simulink model "Longitudinal_U"  (R2024b)
settings: Solver=VariableStepAuto  StartTime=0.0  StopTime=720  RelTol=1e-3
undefined symbols (not defined in the file): Kd_3, Ki_2, Ki_3, Ki_4, Ki_5, Kp_1, Kp_2, Kp_3, Kp_4, Kp_5
libraries: simulink x18, slpidlib x5
settings Model: Creator=GH-X-ST  LastModifiedBy=GH-X-ST

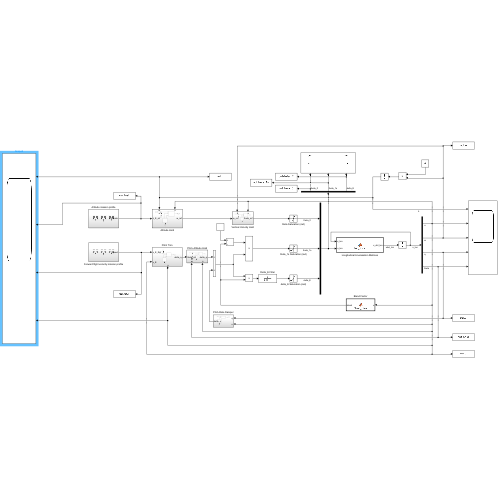
[thumbnail: Simulink's stored preview of the top-level diagram]
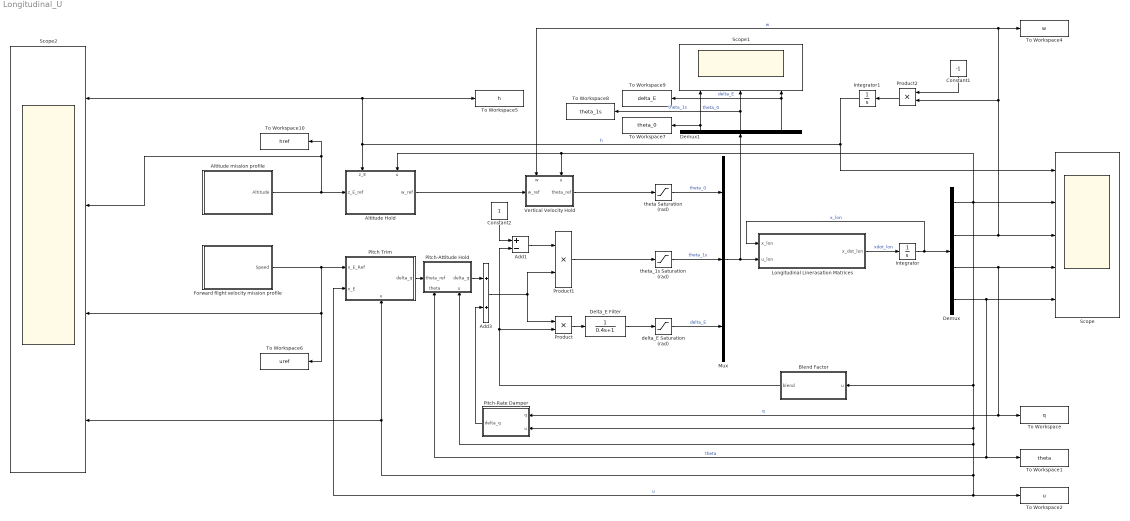
== system Longitudinal_U ==
  Add1 : Sum  Inputs=+-
  Add3 : Sum
  Altitude Hold : Subsystem
      settings: PortSchema="{\"entries\":[{\"content\":{\"sides\":[{\"content\":{\"connectorIds\":[\"In1\"]},\"type\":\"ConnectorPlacement.EquallySpacedRectSide\",\"uuid\":\"786fe27b-9d32-4a4b-ba58-745251b51298\"},{\"content\":{\"connectorIds\":[\"Out1\"],\"side\":\"RIGHT\"},\"type\":\"ConnectorPlacement.EquallySpacedRectSide\",\"uuid\":\"c3e63844-28f7-4108-b9b9-8f5ae49ef2b7\"},{\"content\":{\"connectorIds\":[\"In2\",\"In3\"],\"side\":\"TOP\"},\"type\":\"ConnectorPlacement.EquallySpacedRectSide\",\"uuid\":\"709e7f88-d3c1-4cf0-9a6f-fe71781ed8e6\"}]},\"type\":\"ConnectorPlacement.EquallySpacedConnector\",\"uuid\":\"916bac8a-d735-4a54-bfae-f4eae304bdce\"}],\"packageUris\":[\"http://schema.mathworks.com/mf0/Connector/R2020b\"],\"version\":\"1.0\"}"
  Altitude mission profile : Subsystem
  Blend Factor : MATLAB Function  TreatAsAtomicUnit=on
  Constant1 : Constant  Value=-1
  Constant2 : Constant
  Delta_E Filter : TransferFcn  Denominator=[0.4 1]
  Demux : Demux
  Demux1 : Demux  Outputs=3
  Forward flight velocity mission profile : Subsystem
  Integrator : Integrator  InitialCondition=[0.000000000001; 0; 0; 0]
  Integrator1 : Integrator  InitialCondition=135  ContinuousStateAttributes='h'
  Longitudinal Linerasation Matrices : MATLAB Function  TreatAsAtomicUnit=on
  Mux : Mux  Inputs=3
  Pitch Trim : Subsystem
      settings: PortSchema="{\"entries\":[{\"content\":{\"sides\":[{\"content\":{\"connectorIds\":[\"In1\",\"In2\"]},\"type\":\"ConnectorPlacement.EquallySpacedRectSide\",\"uuid\":\"87058170-54f3-49f3-bbe3-319f98d36a6e\"},{\"content\":{\"connectorIds\":[\"Out1\"],\"side\":\"RIGHT\"},\"type\":\"ConnectorPlacement.EquallySpacedRectSide\",\"uuid\":\"504f7628-6ca7-48d8-902d-2d0a87ee545b\"},{\"content\":{\"side\":\"TOP\"},\"type\":\"ConnectorPlacement.EquallySpacedRectSide\",\"uuid\":\"0adfc2aa-d413-4184-8660-649e124bfc66\"},{\"content\":{\"connectorIds\":[\"In3\"],\"side\":\"BOTTOM\"},\"type\":\"ConnectorPlacement.EquallySpacedRectSide\",\"uuid\":\"db6c614d-9f31-4390-b799-cc5d953a9def\"}]},\"type\":\"ConnectorPlacement.EquallySpacedConnector\",\"uuid\":\"6825786d-d4a2-4d28-866f-fdc5057e89d5\"}],\"packageUris\":[\"http://schema.mathworks.com/mf0/Connector/R2020b\"],\"version\":\"1.0\"}"
  Pitch-Attitude Hold : Subsystem
      settings: PortSchema="{\"entries\":[{\"content\":{\"sides\":[{\"content\":{\"connectorIds\":[\"In1\"]},\"type\":\"ConnectorPlacement.EquallySpacedRectSide\",\"uuid\":\"6ee333b9-9b69-42fd-975a-4580f9624540\"},{\"content\":{\"connectorIds\":[\"Out1\"],\"side\":\"RIGHT\"},\"type\":\"ConnectorPlacement.EquallySpacedRectSide\",\"uuid\":\"6a43d978-a0a5-4636-bfdb-b097e996a039\"},{\"content\":{\"side\":\"TOP\"},\"type\":\"ConnectorPlacement.EquallySpacedRectSide\",\"uuid\":\"00f937d1-ecc9-42d4-adf8-d8f1b79c75a6\"},{\"content\":{\"connectorIds\":[\"In2\",\"In3\"],\"side\":\"BOTTOM\"},\"type\":\"ConnectorPlacement.EquallySpacedRectSide\",\"uuid\":\"809403f9-594f-4491-8a7d-ee0f8643f57e\"}]},\"type\":\"ConnectorPlacement.EquallySpacedConnector\",\"uuid\":\"362aafbc-ebc0-4bb3-8c4e-be284a8bc83f\"}],\"packageUris\":[\"http://schema.mathworks.com/mf0/Connector/R2020b\"],\"version\":\"1.0\"}"
  Pitch-Rate Damper : Subsystem
  Product : Product
  Product1 : Product
  Product2 : Product
  Scope : Scope  NumInputPorts=5
  Scope1 : Scope  NumInputPorts=3
  Scope2 : Scope  NumInputPorts=4
  To Workspace : ToWorkspace  VariableName=q  SaveFormat=Timeseries  SampleTime=-1
  To Workspace1 : ToWorkspace  VariableName=theta  SaveFormat=Timeseries  SampleTime=-1
  To Workspace10 : ToWorkspace  VariableName=href  SaveFormat=Timeseries  SampleTime=-1
  To Workspace2 : ToWorkspace  VariableName=u  SaveFormat=Timeseries  SampleTime=-1
  To Workspace4 : ToWorkspace  VariableName=w  SaveFormat=Timeseries  SampleTime=-1
  To Workspace5 : ToWorkspace  VariableName=h  SaveFormat=Timeseries  SampleTime=-1
  To Workspace6 : ToWorkspace  VariableName=uref  SaveFormat=Timeseries  SampleTime=-1
  To Workspace7 : ToWorkspace  VariableName=theta_0  SaveFormat=Timeseries  SampleTime=-1
  To Workspace8 : ToWorkspace  VariableName=theta_1s  SaveFormat=Timeseries  SampleTime=-1
  To Workspace9 : ToWorkspace  VariableName=delta_E  SaveFormat=Timeseries  SampleTime=-1
  Vertical Velocity Hold : Subsystem
      settings: PortSchema="{\"entries\":[{\"content\":{\"sides\":[{\"content\":{\"connectorIds\":[\"In1\"]},\"type\":\"ConnectorPlacement.EquallySpacedRectSide\",\"uuid\":\"6ee333b9-9b69-42fd-975a-4580f9624540\"},{\"content\":{\"connectorIds\":[\"Out1\"],\"side\":\"RIGHT\"},\"type\":\"ConnectorPlacement.EquallySpacedRectSide\",\"uuid\":\"6a43d978-a0a5-4636-bfdb-b097e996a039\"},{\"content\":{\"connectorIds\":[\"In2\",\"In3\"],\"side\":\"TOP\"},\"type\":\"ConnectorPlacement.EquallySpacedRectSide\",\"uuid\":\"00f937d1-ecc9-42d4-adf8-d8f1b79c75a6\"},{\"content\":{\"side\":\"BOTTOM\"},\"type\":\"ConnectorPlacement.EquallySpacedRectSide\",\"uuid\":\"64d125d6-056c-4640-9df5-5340aaf5f7d1\"}]},\"type\":\"ConnectorPlacement.EquallySpacedConnector\",\"uuid\":\"362aafbc-ebc0-4bb3-8c4e-be284a8bc83f\"}],\"packageUris\":[\"http://schema.mathworks.com/mf0/Connector/R2020b\"],\"version\":\"1.0\"}"
  delta_E Saturation (rad) : Saturate  UpperLimit=deg2rad(11)  LowerLimit=deg2rad(-11)
  theta Saturation (rad) : Saturate  UpperLimit=deg2rad(+20)  LowerLimit=deg2rad(-6)
  theta_1s Saturation (rad) : Saturate  UpperLimit=deg2rad(6)  LowerLimit=deg2rad(-6)
  wires:
  Longitudinal Linerasation Matrices/1(x_dot_lon) -> Integrator/1  "xdot_lon"
  Integrator/1 -> Longitudinal Linerasation Matrices/1(x_lon), Demux/1  "x_lon"
  Demux/1 -> Altitude Hold/3(u), Vertical Velocity Hold/3(u), Scope/2, Blend Factor/1(u), Pitch-Attitude Hold/3(u), Pitch Trim/3(u), Scope2/4, To Workspace2/1, Pitch Trim/2(x_E), Pitch-Rate Damper/2(u)  "u"
  Demux/2 -> Vertical Velocity Hold/2(w), To Workspace4/1, Product2/2, Scope/3  "w"
  Demux/3 -> Scope/4, To Workspace/1, Pitch-Rate Damper/1(q)  "q"
  Demux/4 -> Scope/5, To Workspace1/1, Pitch-Attitude Hold/2(theta)  "theta"
  Blend Factor/1(blend) -> Add1/2, Product/2
  Pitch-Attitude Hold/1(delta_q) -> Add3/1
  Constant2/1 -> Add1/1
  Add1/1 -> Product1/1
  Mux/1 -> Demux1/1, Longitudinal Linerasation Matrices/2(u_lon)
  Demux1/3 -> To Workspace9/1, Scope1/3  "delta_E"
  Demux1/2 -> Scope1/2, To Workspace8/1  "theta_1s"
  Demux1/1 -> Scope1/1, To Workspace7/1  "theta_0"
  Product/1 -> Delta_E Filter/1
  Pitch-Rate Damper/1(delta_q) -> Add3/2
  Constant1/1 -> Product2/1
  Product2/1 -> Integrator1/1
  Integrator1/1 -> Scope/1, Altitude Hold/2(z_E), Scope2/1, To Workspace5/1  "h"
  Altitude Hold/1(w_ref) -> Vertical Velocity Hold/1(w_ref)
  Add3/1 -> Product1/2, Product/1
  Pitch Trim/1(delta_q) -> Pitch-Attitude Hold/1(theta_ref)
  Delta_E Filter/1 -> delta_E Saturation (rad)/1
  delta_E Saturation (rad)/1 -> Mux/3  "delta_E"
  theta_1s Saturation (rad)/1 -> Mux/2  "theta_1s"
  Product1/1 -> theta_1s Saturation (rad)/1
  Vertical Velocity Hold/1(theta_ref) -> theta Saturation (rad)/1
  theta Saturation (rad)/1 -> Mux/1  "theta_0"
  Altitude mission profile/1(Altitude) -> To Workspace10/1, Scope2/2, Altitude Hold/1(z_E_ref)
  Forward flight velocity mission profile/1(Speed) -> To Workspace6/1, Scope2/3, Pitch Trim/1(x_E_Ref)

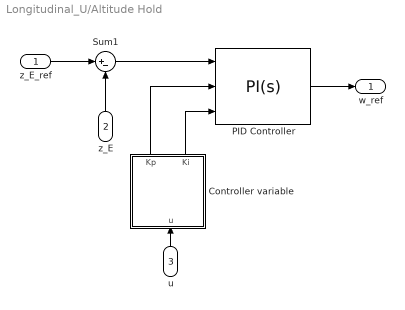
== system Longitudinal_U/Altitude Hold ==
  z_E_ref : Inport
  z_E : Inport  Port=2
  u : Inport  Port=3
  Controller variable : MATLAB Function  TreatAsAtomicUnit=on
  PID Controller : slpidlib/PID Controller  Controller=PI  Form=Parallel  TimeDomain=Continuous-time  UseExternalTs=off  SampleTime=-1  IntegratorMethod=Forward Euler  FilterMethod=Forward Euler  ControllerParametersSource=external  P=Kp_5  I=Ki_5  UseKiTs=off  D=0.005  UseExternalDerivativeSource=off  N=100  UseFilter=on  TunerSelectOption=Transfer Function Based (PID Tuner App)  InitialConditionSource=internal  InitialConditionForIntegrator=0  InitialConditionForFilter=0  DifferentiatorICPrevScaledInput=0  ExternalReset=none  TrackingMode=off  Kt=1  LimitOutput=on  SatLimitsSource=internal  UpperSaturationLimit=1  LowerSaturationLimit=-1  LinearizeAsGain=on  AntiWindupMode=none  Kb=1  LimitIntegrator=off  UpperIntegratorSaturationLimit=inf  LowerIntegratorSaturationLimit=-inf  POutMin=[]  POutMax=[]  IOutMin=[]  IOutMax=[]  DOutMin=[]  DOutMax=[]  NOutMin=[]  NOutMax=[]  SumOutMin=[]  SumOutMax=[]  SaturationOutMin=[]  SaturationOutMax=[]  PParamMin=[]  PParamMax=[]  IParamMin=[]  IParamMax=[]  DParamMin=[]  DParamMax=[]  NParamMin=[]  NParamMax=[]  KbParamMin=[]  KbParamMax=[]  KtParamMin=[]  KtParamMax=[]  KbOutMin=[]  KbOutMax=[]  KtOutMin=[]  KtOutMax=[]  IntegratorOutMin=[]  IntegratorOutMax=[]  FilterOutMin=[]  FilterOutMax=[]  SumI1OutMin=[]  SumI1OutMax=[]  SumI2OutMin=[]  SumI2OutMax=[]  SumI3OutMin=[]  SumI3OutMax=[]  SumI4OutMin=[]  SumI4OutMax=[]  SumDOutMin=[]  SumDOutMax=[]  DifferentiatorOutMin=[]  DifferentiatorOutMax=[]  FilterDiffOutCoefMin=[]  FilterDiffOutCoefMax=[]  ReciprocalOutMin=[]  ReciprocalOutMax=[]  SumDenOutMin=[]  SumDenOutMax=[]  SumNumOutMin=[]  SumNumOutMax=[]  DivideOutMin=[]  DivideOutMax=[]  UdiffTsProdOutMin=[]  UdiffTsProdOutMax=[]  NTsProdOutMin=[]  NTsProdOutMax=[]  UintegralTsProdOutMin=[]  UintegralTsProdOutMax=[]  UngainTsProdOutMin=[]  UngainTsProdOutMax=[]  ClampingZeroOutDataTypeStr=Inherit: Inherit via back propagation  ClampingZeroOutMin=[]  ClampingZeroOutMax=[]  FilterDenConstantOutDataTypeStr=Inherit: Inherit via back propagation  FilterDenConstantOutMin=[]  FilterDenConstantOutMax=[]  PCopyOutDataTypeStr=Inherit: Inherit via back propagation  PCopyOutMin=[]  PCopyOutMax=[]  NCopyOutDataTypeStr=Inherit: Inherit via back propagation  NCopyOutMin=[]  NCopyOutMax=[]  IntegratorContinuousStateAttributes=''  IntegratorStateMustResolveToSignalObject=off  IntegratorRTWStateStorageClass=Auto  FilterContinuousStateAttributes=''  FilterStateMustResolveToSignalObject=off  FilterRTWStateStorageClass=Auto  ParallelPVariant=ExternalParameters  IdealPVariant=Disabled  IVariant=ExternalParameters  DVariant=Disabled  IntegratorVariant=Continuous  SatVariant=Enabled  AWVariant=Passthrough  PCopyVariant=Disabled  TRVariant=Disabled  FdbkBlocksVariant=Forward  IdealPFdbkVariant=Disabled  SatFdbkVariant=Disabled  DerivativeFilterVariant=Disabled  NVariant=Disabled  NCopyVariant=Disabled_SignalSpec  FilterICVariant=Disabled  IntegratorICVariant=InternalICs  ExternalResetVariant=Disabled  TRSumVariant=Passthrough  SumFdbkVariant=Disabled  SumVariant=Sum_PI  TsampFilterVariant=InternalTs  TsampNgainVariant=Passthrough  TsampIntegralVariant=Disabled_SignalSpec  ExternalSaturationOutDataTypeStr=Inherit: Same as second input  DerivativeSourceVariant=Disabled  PreIntVariant=InternalPreInt
  Sum1 : Sum  Inputs=|+-
  w_ref : Outport
  wires:
  PID Controller/1 -> w_ref/1
  Sum1/1 -> PID Controller/1
  z_E_ref/1 -> Sum1/1
  z_E/1 -> Sum1/2
  u/1 -> Controller variable/1(u)
  Controller variable/1(Kp) -> PID Controller/2
  Controller variable/2(Ki) -> PID Controller/3

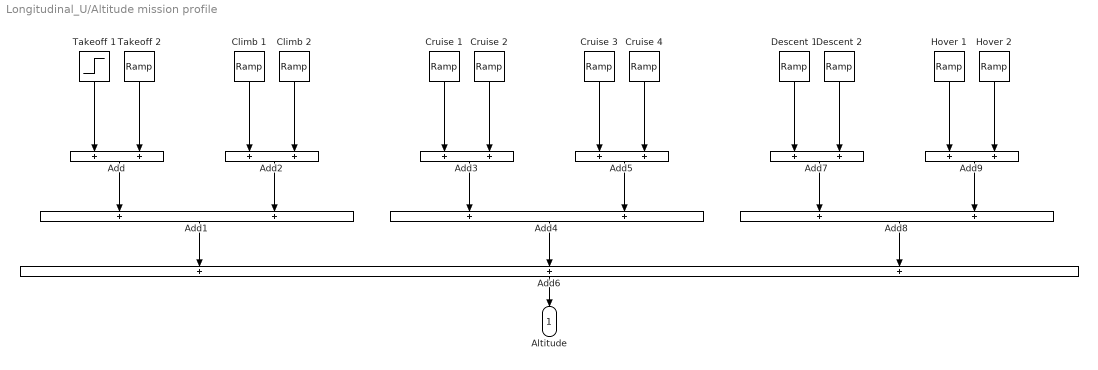
== system Longitudinal_U/Altitude mission profile ==
  Add{,1..5,7..9} (9 alike) : Sum
  Add6 : Sum  Inputs=+++
  Climb 1 : simulink/Sources/Ramp  slope=0.4  start=50  InitialOutput=0
  Climb 2 : simulink/Sources/Ramp  slope=-0.4  start=100  InitialOutput=0
  Cruise 1 : simulink/Sources/Ramp  slope=0.1  start=100  InitialOutput=0
  Cruise 2 : simulink/Sources/Ramp  slope=-0.1  start=200  InitialOutput=0
  Cruise 3 : simulink/Sources/Ramp  slope=0  start=200  InitialOutput=0
  Cruise 4 : simulink/Sources/Ramp  slope=0  start=350  InitialOutput=0
  Descent 1 : simulink/Sources/Ramp  slope=-12/70  start=350  InitialOutput=0
  Descent 2 : simulink/Sources/Ramp  slope=12/70  start=475  InitialOutput=0
  Hover 1 : simulink/Sources/Ramp  slope=0  start=475  InitialOutput=0
  Hover 2 : simulink/Sources/Ramp  slope=0  start=600  InitialOutput=0
  Takeoff 1 : Step  Time=0  Before=135  After=150  SampleTime=0
  Takeoff 2 : simulink/Sources/Ramp  slope=0  start=50  InitialOutput=0
  Altitude : Outport
  wires:
  Add1/1 -> Add6/1
  Climb 2/1 -> Add2/2
  Add4/1 -> Add6/2
  Climb 1/1 -> Add2/1
  Hover 1/1 -> Add9/1
  Add7/1 -> Add8/1
  Descent 1/1 -> Add7/1
  Add9/1 -> Add8/2
  Hover 2/1 -> Add9/2
  Add8/1 -> Add6/3
  Add2/1 -> Add1/2
  Add3/1 -> Add4/1
  Add5/1 -> Add4/2
  Cruise 2/1 -> Add3/2
  Cruise 4/1 -> Add5/2
  Cruise 1/1 -> Add3/1
  Cruise 3/1 -> Add5/1
  Descent 2/1 -> Add7/2
  Takeoff 2/1 -> Add/2
  Takeoff 1/1 -> Add/1
  Add/1 -> Add1/1
  Add6/1 -> Altitude/1

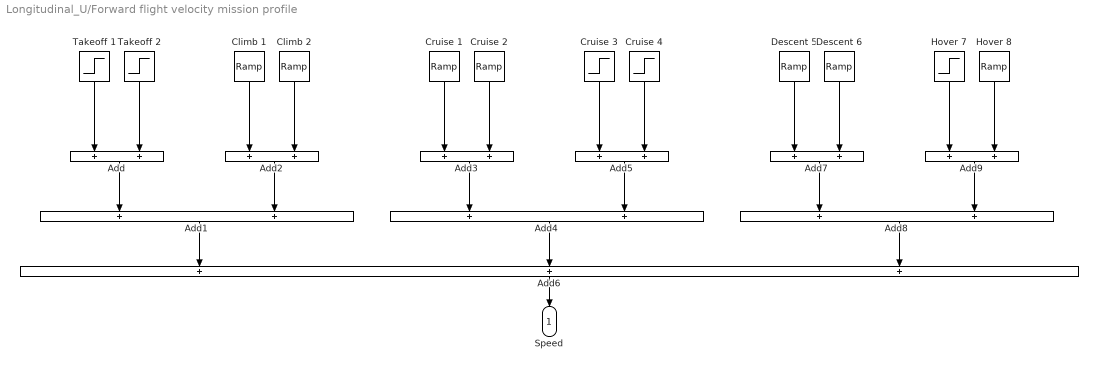
== system Longitudinal_U/Forward flight velocity mission profile ==
  Add{,1..5,7..9} (9 alike) : Sum
  Add6 : Sum  Inputs=+++
  Climb 1 : simulink/Sources/Ramp  slope=0.4  start=50  InitialOutput=0
  Climb 2 : simulink/Sources/Ramp  slope=-0.4  start=100  InitialOutput=0
  Cruise 1 : simulink/Sources/Ramp  slope=0  start=100  InitialOutput=0
  Cruise 2 : simulink/Sources/Ramp  slope=0  start=200  InitialOutput=0
  Cruise 3 : Step  Time=200  After=22  SampleTime=0
  Cruise 4 : Step  Time=350  After=-37  SampleTime=0
  Descent 5 : simulink/Sources/Ramp  slope=0  start=350  InitialOutput=0
  Descent 6 : simulink/Sources/Ramp  slope=0  start=475  InitialOutput=0
  Hover 7 : Step  Time=475  After=-35  SampleTime=0
  Hover 8 : simulink/Sources/Ramp  slope=0  start=600  InitialOutput=0
  Takeoff 1 : Step  Time=0  After=0  SampleTime=0
  Takeoff 2 : Step  Time=50  After=30  SampleTime=0
  Speed : Outport
  wires:
  Add6/1 -> Speed/1
  Add1/1 -> Add6/1
  Climb 2/1 -> Add2/2
  Add4/1 -> Add6/2
  Climb 1/1 -> Add2/1
  Add7/1 -> Add8/1
  Descent 5/1 -> Add7/1
  Add9/1 -> Add8/2
  Descent 6/1 -> Add7/2
  Hover 8/1 -> Add9/2
  Add8/1 -> Add6/3
  Add2/1 -> Add1/2
  Add3/1 -> Add4/1
  Add5/1 -> Add4/2
  Cruise 1/1 -> Add3/1
  Cruise 4/1 -> Add5/2
  Add/1 -> Add1/1
  Hover 7/1 -> Add9/1
  Takeoff 1/1 -> Add/1
  Takeoff 2/1 -> Add/2
  Cruise 3/1 -> Add5/1
  Cruise 2/1 -> Add3/2

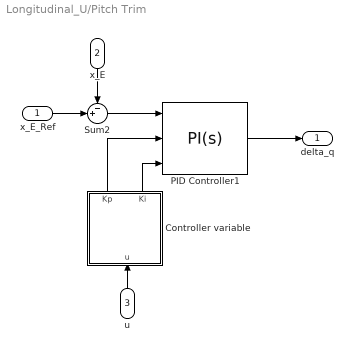
== system Longitudinal_U/Pitch Trim ==
  x_E_Ref : Inport
  x_E : Inport  Port=2
  u : Inport  Port=3
  Controller variable : MATLAB Function  TreatAsAtomicUnit=on
  PID Controller1 : slpidlib/PID Controller  Controller=PI  Form=Parallel  TimeDomain=Continuous-time  UseExternalTs=off  SampleTime=-1  IntegratorMethod=Forward Euler  FilterMethod=Forward Euler  ControllerParametersSource=external  P=Kp_3  I=Ki_3  UseKiTs=off  D=Kd_3  UseExternalDerivativeSource=off  N=100  UseFilter=on  TunerSelectOption=Transfer Function Based (PID Tuner App)  InitialConditionSource=internal  InitialConditionForIntegrator=0  InitialConditionForFilter=0  DifferentiatorICPrevScaledInput=0  ExternalReset=none  TrackingMode=off  Kt=1  LimitOutput=on  SatLimitsSource=internal  UpperSaturationLimit=1  LowerSaturationLimit=-1  LinearizeAsGain=on  AntiWindupMode=none  Kb=1  LimitIntegrator=off  UpperIntegratorSaturationLimit=inf  LowerIntegratorSaturationLimit=-inf  POutMin=[]  POutMax=[]  IOutMin=[]  IOutMax=[]  DOutMin=[]  DOutMax=[]  NOutMin=[]  NOutMax=[]  SumOutMin=[]  SumOutMax=[]  SaturationOutMin=[]  SaturationOutMax=[]  PParamMin=[]  PParamMax=[]  IParamMin=[]  IParamMax=[]  DParamMin=[]  DParamMax=[]  NParamMin=[]  NParamMax=[]  KbParamMin=[]  KbParamMax=[]  KtParamMin=[]  KtParamMax=[]  KbOutMin=[]  KbOutMax=[]  KtOutMin=[]  KtOutMax=[]  IntegratorOutMin=[]  IntegratorOutMax=[]  FilterOutMin=[]  FilterOutMax=[]  SumI1OutMin=[]  SumI1OutMax=[]  SumI2OutMin=[]  SumI2OutMax=[]  SumI3OutMin=[]  SumI3OutMax=[]  SumI4OutMin=[]  SumI4OutMax=[]  SumDOutMin=[]  SumDOutMax=[]  DifferentiatorOutMin=[]  DifferentiatorOutMax=[]  FilterDiffOutCoefMin=[]  FilterDiffOutCoefMax=[]  ReciprocalOutMin=[]  ReciprocalOutMax=[]  SumDenOutMin=[]  SumDenOutMax=[]  SumNumOutMin=[]  SumNumOutMax=[]  DivideOutMin=[]  DivideOutMax=[]  UdiffTsProdOutMin=[]  UdiffTsProdOutMax=[]  NTsProdOutMin=[]  NTsProdOutMax=[]  UintegralTsProdOutMin=[]  UintegralTsProdOutMax=[]  UngainTsProdOutMin=[]  UngainTsProdOutMax=[]  ClampingZeroOutDataTypeStr=Inherit: Inherit via back propagation  ClampingZeroOutMin=[]  ClampingZeroOutMax=[]  FilterDenConstantOutDataTypeStr=Inherit: Inherit via back propagation  FilterDenConstantOutMin=[]  FilterDenConstantOutMax=[]  PCopyOutDataTypeStr=Inherit: Inherit via back propagation  PCopyOutMin=[]  PCopyOutMax=[]  NCopyOutDataTypeStr=Inherit: Inherit via back propagation  NCopyOutMin=[]  NCopyOutMax=[]  IntegratorContinuousStateAttributes=''  IntegratorStateMustResolveToSignalObject=off  IntegratorRTWStateStorageClass=Auto  FilterContinuousStateAttributes=''  FilterStateMustResolveToSignalObject=off  FilterRTWStateStorageClass=Auto  ParallelPVariant=ExternalParameters  IdealPVariant=Disabled  IVariant=ExternalParameters  DVariant=Disabled  IntegratorVariant=Continuous  SatVariant=Enabled  AWVariant=Passthrough  PCopyVariant=Disabled  TRVariant=Disabled  FdbkBlocksVariant=Forward  IdealPFdbkVariant=Disabled  SatFdbkVariant=Disabled  DerivativeFilterVariant=Disabled  NVariant=Disabled  NCopyVariant=Disabled_SignalSpec  FilterICVariant=Disabled  IntegratorICVariant=InternalICs  ExternalResetVariant=Disabled  TRSumVariant=Passthrough  SumFdbkVariant=Disabled  SumVariant=Sum_PI  TsampFilterVariant=InternalTs  TsampNgainVariant=Passthrough  TsampIntegralVariant=Disabled_SignalSpec  ExternalSaturationOutDataTypeStr=Inherit: Same as second input  DerivativeSourceVariant=Disabled  PreIntVariant=InternalPreInt
  Sum2 : Sum  Inputs=-+|
  delta_q : Outport
  wires:
  x_E/1 -> Sum2/1
  x_E_Ref/1 -> Sum2/2
  PID Controller1/1 -> delta_q/1
  Sum2/1 -> PID Controller1/1
  u/1 -> Controller variable/1(u)
  Controller variable/1(Kp) -> PID Controller1/2
  Controller variable/2(Ki) -> PID Controller1/3

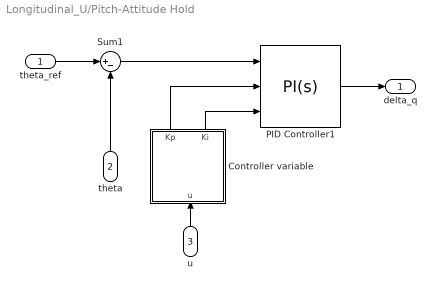
== system Longitudinal_U/Pitch-Attitude Hold ==
  theta_ref : Inport
  theta : Inport  Port=2
  u : Inport  Port=3
  Controller variable : MATLAB Function  TreatAsAtomicUnit=on
  PID Controller1 : slpidlib/PID Controller  Controller=PI  Form=Parallel  TimeDomain=Continuous-time  UseExternalTs=off  SampleTime=-1  IntegratorMethod=Forward Euler  FilterMethod=Forward Euler  ControllerParametersSource=external  P=Kp_2  I=Ki_2  UseKiTs=off  D=0.005  UseExternalDerivativeSource=on  N=100  UseFilter=on  TunerSelectOption=Transfer Function Based (PID Tuner App)  InitialConditionSource=internal  InitialConditionForIntegrator=0  InitialConditionForFilter=0  DifferentiatorICPrevScaledInput=0  ExternalReset=none  TrackingMode=off  Kt=1  LimitOutput=on  SatLimitsSource=internal  UpperSaturationLimit=1  LowerSaturationLimit=-1  LinearizeAsGain=on  AntiWindupMode=none  Kb=1  LimitIntegrator=off  UpperIntegratorSaturationLimit=inf  LowerIntegratorSaturationLimit=-inf  POutMin=[]  POutMax=[]  IOutMin=[]  IOutMax=[]  DOutMin=[]  DOutMax=[]  NOutMin=[]  NOutMax=[]  SumOutMin=[]  SumOutMax=[]  SaturationOutMin=[]  SaturationOutMax=[]  PParamMin=[]  PParamMax=[]  IParamMin=[]  IParamMax=[]  DParamMin=[]  DParamMax=[]  NParamMin=[]  NParamMax=[]  KbParamMin=[]  KbParamMax=[]  KtParamMin=[]  KtParamMax=[]  KbOutMin=[]  KbOutMax=[]  KtOutMin=[]  KtOutMax=[]  IntegratorOutMin=[]  IntegratorOutMax=[]  FilterOutMin=[]  FilterOutMax=[]  SumI1OutMin=[]  SumI1OutMax=[]  SumI2OutMin=[]  SumI2OutMax=[]  SumI3OutMin=[]  SumI3OutMax=[]  SumI4OutMin=[]  SumI4OutMax=[]  SumDOutMin=[]  SumDOutMax=[]  DifferentiatorOutMin=[]  DifferentiatorOutMax=[]  FilterDiffOutCoefMin=[]  FilterDiffOutCoefMax=[]  ReciprocalOutMin=[]  ReciprocalOutMax=[]  SumDenOutMin=[]  SumDenOutMax=[]  SumNumOutMin=[]  SumNumOutMax=[]  DivideOutMin=[]  DivideOutMax=[]  UdiffTsProdOutMin=[]  UdiffTsProdOutMax=[]  NTsProdOutMin=[]  NTsProdOutMax=[]  UintegralTsProdOutMin=[]  UintegralTsProdOutMax=[]  UngainTsProdOutMin=[]  UngainTsProdOutMax=[]  ClampingZeroOutDataTypeStr=Inherit: Inherit via back propagation  ClampingZeroOutMin=[]  ClampingZeroOutMax=[]  FilterDenConstantOutDataTypeStr=Inherit: Inherit via back propagation  FilterDenConstantOutMin=[]  FilterDenConstantOutMax=[]  PCopyOutDataTypeStr=Inherit: Inherit via back propagation  PCopyOutMin=[]  PCopyOutMax=[]  NCopyOutDataTypeStr=Inherit: Inherit via back propagation  NCopyOutMin=[]  NCopyOutMax=[]  IntegratorContinuousStateAttributes=''  IntegratorStateMustResolveToSignalObject=off  IntegratorRTWStateStorageClass=Auto  FilterContinuousStateAttributes=''  FilterStateMustResolveToSignalObject=off  FilterRTWStateStorageClass=Auto  ParallelPVariant=ExternalParameters  IdealPVariant=Disabled  IVariant=ExternalParameters  DVariant=Disabled  IntegratorVariant=Continuous  SatVariant=Enabled  AWVariant=Passthrough  PCopyVariant=Disabled  TRVariant=Disabled  FdbkBlocksVariant=Forward  IdealPFdbkVariant=Disabled  SatFdbkVariant=Disabled  DerivativeFilterVariant=Disabled  NVariant=Passthrough  NCopyVariant=Disabled_SignalSpec  FilterICVariant=Disabled  IntegratorICVariant=InternalICs  ExternalResetVariant=Disabled  TRSumVariant=Passthrough  SumFdbkVariant=Disabled  SumVariant=Sum_PI  TsampFilterVariant=InternalTs  TsampNgainVariant=Passthrough  TsampIntegralVariant=Disabled_SignalSpec  ExternalSaturationOutDataTypeStr=Inherit: Same as second input  DerivativeSourceVariant=Disabled  PreIntVariant=InternalPreInt
  Sum1 : Sum  Inputs=|+-
  delta_q : Outport
  wires:
  PID Controller1/1 -> delta_q/1
  theta_ref/1 -> Sum1/1
  theta/1 -> Sum1/2
  Sum1/1 -> PID Controller1/1
  Controller variable/1(Kp) -> PID Controller1/2
  Controller variable/2(Ki) -> PID Controller1/3
  u/1 -> Controller variable/1(u)

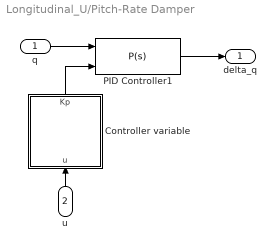
== system Longitudinal_U/Pitch-Rate Damper ==
  q : Inport
  u : Inport  Port=2
  Controller variable : MATLAB Function  TreatAsAtomicUnit=on
  PID Controller1 : slpidlib/PID Controller  Controller=P  Form=Parallel  TimeDomain=Continuous-time  UseExternalTs=off  SampleTime=-1  IntegratorMethod=Forward Euler  FilterMethod=Forward Euler  ControllerParametersSource=external  P=Kp_1  I=0.005  UseKiTs=off  D=0.005  UseExternalDerivativeSource=on  N=100  UseFilter=on  TunerSelectOption=Transfer Function Based (PID Tuner App)  InitialConditionSource=internal  InitialConditionForIntegrator=0  InitialConditionForFilter=0  DifferentiatorICPrevScaledInput=0  ExternalReset=none  TrackingMode=off  Kt=1  LimitOutput=on  SatLimitsSource=internal  UpperSaturationLimit=1  LowerSaturationLimit=-1  LinearizeAsGain=on  AntiWindupMode=none  Kb=1  LimitIntegrator=off  UpperIntegratorSaturationLimit=inf  LowerIntegratorSaturationLimit=-inf  POutMin=[]  POutMax=[]  IOutMin=[]  IOutMax=[]  DOutMin=[]  DOutMax=[]  NOutMin=[]  NOutMax=[]  SumOutMin=[]  SumOutMax=[]  SaturationOutMin=[]  SaturationOutMax=[]  PParamMin=[]  PParamMax=[]  IParamMin=[]  IParamMax=[]  DParamMin=[]  DParamMax=[]  NParamMin=[]  NParamMax=[]  KbParamMin=[]  KbParamMax=[]  KtParamMin=[]  KtParamMax=[]  KbOutMin=[]  KbOutMax=[]  KtOutMin=[]  KtOutMax=[]  IntegratorOutMin=[]  IntegratorOutMax=[]  FilterOutMin=[]  FilterOutMax=[]  SumI1OutMin=[]  SumI1OutMax=[]  SumI2OutMin=[]  SumI2OutMax=[]  SumI3OutMin=[]  SumI3OutMax=[]  SumI4OutMin=[]  SumI4OutMax=[]  SumDOutMin=[]  SumDOutMax=[]  DifferentiatorOutMin=[]  DifferentiatorOutMax=[]  FilterDiffOutCoefMin=[]  FilterDiffOutCoefMax=[]  ReciprocalOutMin=[]  ReciprocalOutMax=[]  SumDenOutMin=[]  SumDenOutMax=[]  SumNumOutMin=[]  SumNumOutMax=[]  DivideOutMin=[]  DivideOutMax=[]  UdiffTsProdOutMin=[]  UdiffTsProdOutMax=[]  NTsProdOutMin=[]  NTsProdOutMax=[]  UintegralTsProdOutMin=[]  UintegralTsProdOutMax=[]  UngainTsProdOutMin=[]  UngainTsProdOutMax=[]  ClampingZeroOutDataTypeStr=Inherit: Inherit via back propagation  ClampingZeroOutMin=[]  ClampingZeroOutMax=[]  FilterDenConstantOutDataTypeStr=Inherit: Inherit via back propagation  FilterDenConstantOutMin=[]  FilterDenConstantOutMax=[]  PCopyOutDataTypeStr=Inherit: Inherit via back propagation  PCopyOutMin=[]  PCopyOutMax=[]  NCopyOutDataTypeStr=Inherit: Inherit via back propagation  NCopyOutMin=[]  NCopyOutMax=[]  IntegratorContinuousStateAttributes=''  IntegratorStateMustResolveToSignalObject=off  IntegratorRTWStateStorageClass=Auto  FilterContinuousStateAttributes=''  FilterStateMustResolveToSignalObject=off  FilterRTWStateStorageClass=Auto  ParallelPVariant=ExternalParameters  IdealPVariant=Disabled  IVariant=Disabled  DVariant=Disabled  IntegratorVariant=Disabled  SatVariant=Enabled  AWVariant=Disabled  PCopyVariant=Disabled  TRVariant=Disabled  FdbkBlocksVariant=Forward  IdealPFdbkVariant=Disabled  SatFdbkVariant=Disabled  DerivativeFilterVariant=Disabled  NVariant=Passthrough  NCopyVariant=Disabled_SignalSpec  FilterICVariant=Disabled  IntegratorICVariant=Disabled  ExternalResetVariant=Disabled  TRSumVariant=Passthrough  SumFdbkVariant=Disabled  SumVariant=Passthrough_P  TsampFilterVariant=InternalTs  TsampNgainVariant=Passthrough  TsampIntegralVariant=Disabled_SignalSpec  ExternalSaturationOutDataTypeStr=Inherit: Same as second input  DerivativeSourceVariant=Disabled  PreIntVariant=InternalPreInt
  delta_q : Outport
  wires:
  PID Controller1/1 -> delta_q/1
  q/1 -> PID Controller1/1
  Controller variable/1(Kp) -> PID Controller1/2
  u/1 -> Controller variable/1(u)

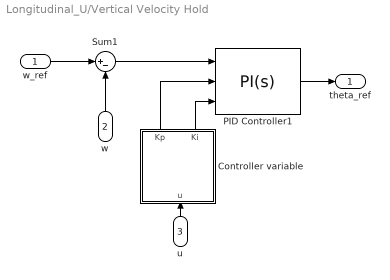
== system Longitudinal_U/Vertical Velocity Hold ==
  w_ref : Inport
  w : Inport  Port=2
  u : Inport  Port=3
  Controller variable : MATLAB Function  TreatAsAtomicUnit=on
  PID Controller1 : slpidlib/PID Controller  Controller=PI  Form=Parallel  TimeDomain=Continuous-time  UseExternalTs=off  SampleTime=-1  IntegratorMethod=Forward Euler  FilterMethod=Forward Euler  ControllerParametersSource=external  P=Kp_4  I=Ki_4  UseKiTs=off  D=0.005  UseExternalDerivativeSource=on  N=100  UseFilter=on  TunerSelectOption=Transfer Function Based (PID Tuner App)  InitialConditionSource=internal  InitialConditionForIntegrator=0  InitialConditionForFilter=0  DifferentiatorICPrevScaledInput=0  ExternalReset=none  TrackingMode=off  Kt=1  LimitOutput=on  SatLimitsSource=internal  UpperSaturationLimit=1  LowerSaturationLimit=-1  LinearizeAsGain=on  AntiWindupMode=none  Kb=1  LimitIntegrator=off  UpperIntegratorSaturationLimit=inf  LowerIntegratorSaturationLimit=-inf  POutMin=[]  POutMax=[]  IOutMin=[]  IOutMax=[]  DOutMin=[]  DOutMax=[]  NOutMin=[]  NOutMax=[]  SumOutMin=[]  SumOutMax=[]  SaturationOutMin=[]  SaturationOutMax=[]  PParamMin=[]  PParamMax=[]  IParamMin=[]  IParamMax=[]  DParamMin=[]  DParamMax=[]  NParamMin=[]  NParamMax=[]  KbParamMin=[]  KbParamMax=[]  KtParamMin=[]  KtParamMax=[]  KbOutMin=[]  KbOutMax=[]  KtOutMin=[]  KtOutMax=[]  IntegratorOutMin=[]  IntegratorOutMax=[]  FilterOutMin=[]  FilterOutMax=[]  SumI1OutMin=[]  SumI1OutMax=[]  SumI2OutMin=[]  SumI2OutMax=[]  SumI3OutMin=[]  SumI3OutMax=[]  SumI4OutMin=[]  SumI4OutMax=[]  SumDOutMin=[]  SumDOutMax=[]  DifferentiatorOutMin=[]  DifferentiatorOutMax=[]  FilterDiffOutCoefMin=[]  FilterDiffOutCoefMax=[]  ReciprocalOutMin=[]  ReciprocalOutMax=[]  SumDenOutMin=[]  SumDenOutMax=[]  SumNumOutMin=[]  SumNumOutMax=[]  DivideOutMin=[]  DivideOutMax=[]  UdiffTsProdOutMin=[]  UdiffTsProdOutMax=[]  NTsProdOutMin=[]  NTsProdOutMax=[]  UintegralTsProdOutMin=[]  UintegralTsProdOutMax=[]  UngainTsProdOutMin=[]  UngainTsProdOutMax=[]  ClampingZeroOutDataTypeStr=Inherit: Inherit via back propagation  ClampingZeroOutMin=[]  ClampingZeroOutMax=[]  FilterDenConstantOutDataTypeStr=Inherit: Inherit via back propagation  FilterDenConstantOutMin=[]  FilterDenConstantOutMax=[]  PCopyOutDataTypeStr=Inherit: Inherit via back propagation  PCopyOutMin=[]  PCopyOutMax=[]  NCopyOutDataTypeStr=Inherit: Inherit via back propagation  NCopyOutMin=[]  NCopyOutMax=[]  IntegratorContinuousStateAttributes=''  IntegratorStateMustResolveToSignalObject=off  IntegratorRTWStateStorageClass=Auto  FilterContinuousStateAttributes=''  FilterStateMustResolveToSignalObject=off  FilterRTWStateStorageClass=Auto  ParallelPVariant=ExternalParameters  IdealPVariant=Disabled  IVariant=ExternalParameters  DVariant=Disabled  IntegratorVariant=Continuous  SatVariant=Enabled  AWVariant=Passthrough  PCopyVariant=Disabled  TRVariant=Disabled  FdbkBlocksVariant=Forward  IdealPFdbkVariant=Disabled  SatFdbkVariant=Disabled  DerivativeFilterVariant=Disabled  NVariant=Passthrough  NCopyVariant=Disabled_SignalSpec  FilterICVariant=Disabled  IntegratorICVariant=InternalICs  ExternalResetVariant=Disabled  TRSumVariant=Passthrough  SumFdbkVariant=Disabled  SumVariant=Sum_PI  TsampFilterVariant=InternalTs  TsampNgainVariant=Passthrough  TsampIntegralVariant=Disabled_SignalSpec  ExternalSaturationOutDataTypeStr=Inherit: Same as second input  DerivativeSourceVariant=Disabled  PreIntVariant=InternalPreInt
  Sum1 : Sum  Inputs=|+-
  theta_ref : Outport
  wires:
  PID Controller1/1 -> theta_ref/1
  Sum1/1 -> PID Controller1/1
  w_ref/1 -> Sum1/1
  w/1 -> Sum1/2
  u/1 -> Controller variable/1(u)
  Controller variable/1(Kp) -> PID Controller1/2
  Controller variable/2(Ki) -> PID Controller1/3

== matlab function Longitudinal_U/Pitch-Rate Damper/Controller variable ==
  data: Kp output; u input
function Kp = Find_K1(u)
% Author:
%   Hanchen Li (hl3422@ic.ac.uk)
%
% Inputs:
%   u         - Forward velocity (m/s)
%
% Outputs:
%  Kp

U = [10.01; 20; 40; 60; 72.0222222];

if abs(u) <= 40

    Kp = 25.3;

else

    u = abs(u);
    u = min(max(u, min(U)), max(U));
    
    Kp_s = [97.0 84.1 25.3 9.65 7.80];
    
    Kp =  interp1(U, Kp_s, u, 'pchip', 'extrap');
    
end

end

== matlab function Longitudinal_U/Longitudinal Linerasation Matrices ==
  data: x_lon input; u_lon input; x_dot_lon output
function x_dot_lon = Lon_linear(x_lon, u_lon)
% Author:
%   Hanchen Li (hl3422@ic.ac.uk)
%
% Inputs:
%   x_lon     - [u, w, q, theta]
%   u         - Forward velocity (m/s)
%   w         - Vertical velocity (m/s)
%   q         - Pitch rate (rad/s)
%   theta     - Euler pitch angle (rad)
%
%   u_lon     - [theta_0, theta_1s, delta_E]
%   theta_0   - Average rotor collective (rad)
%   theta_1s  - Longitudinal cyclic (rad)
%   delta_E   - Elevator deflection (rad)
%
% Outputs:
%   x_dot_lon - [u_dot, w_dot, q_dot, theta_dot]

%% 0 Extract Parameters
u     = x_lon(1);
% w     = x_lon(2);
% q     = x_lon(3);
% theta = x_lon(4);

% theta_0 = u_lon(1);
% theta_1s = u_lon(2);
% delta_E = u_lon(3);

%%  1 Initial parameters
U = [10.01; 20; 40; 60; 72.0222222];       % 5 break-points

A_lon_all = cat(3,...
[0.00797773730409901	0.0742775144324526	-1.21387619054530	-9.79666335749863;
-0.300981219236718	-1.37899711980971	10.9535968552343	-0.454094238238056;
0.0867879507802988	0.0518221856357636	-1.66200207187276	0;
0	0	0.999987703616044	0],...
[-0.0112549858980772	0.0371668055628924	-1.18927896465665	-9.80422222650819;
-0.133476123611587	-1.29584894245305	20.8981012783838	-0.0361550902372443;
0.0229512851532743	0.0212311520956117	-1.57834195971935	0;
0	0	0.999823172370649	0],...
[-0.00894644618554263	0.0320555490226915	-1.19654303458228	-9.78886874671681;
0.0177938328871363	-2.75625714952099	41.9669994347238	0.0565348232672847;
0.00544480361520019	0.0390031290231026	-1.68547625422026	0;
0	0	0.999701937133157	0],...
[-0.00115522776185373	0.0138477446845475	-1.25249222634898	-9.78189512322418;
0.129681745697496	-2.84658770249635	62.0992998719228	-0.370385725787514;
-6.84962619262734e-05	0.0554454638454316	-1.71412794300992	0;
0	0	0.999829013944947	0],...
[0.00198907487199834	0.00124807180451603	-1.31545814391634	-9.77936080280246;
0.208959151679622	-2.91377790533787	74.4525040940847	-0.690902155824347;
-0.00261903529268842	0.0663122914709030	-1.76288467057787	0;
0	0	0.999876306745786	0]);

B_lon_all = cat(3,...
[10.6236577255089	-7.56754553412536	0.00130717492913268;
-223.536674937179	-16.2402084532332	-0.180124033315465;
-2.09157792284219	-17.4158153969991	-0.0756279848803381;
0	0	0],...
[3.61243491647048	-7.51807669482774	0.00519991275444581;
-211.546063860615	-28.3860279697912	-0.718873847311841;
-3.72624202744466	-15.9950728844985	-0.301829974738856;
0	0	0],...
[-2.10906781602821	-8.34051477693776	-0.000966485101117076;
-228.851268194816	-60.5903363544424	-2.65783402805475;
-7.49489399091787	-17.9234263896394	-1.11495618916578;
0	0	0],...
[-6.26132311908841	-9.73615029140097	0;
-245.122010910137	-92.4433695878246	-6.00187247789208;
-13.3651657046107	-20.4991398778183	-2.51787921575724;
0	0	0],...
[-9.36734534820370	-11.2809889940346	0;
-257.948569477389	-112.985439522211	-8.64803218389554;
-16.7725921688728	-22.1441400308729	-3.62798452869815;
0	0	0]);


%% 2  Vectorised interpolation
method = 'pchip';

% permute ->  (break-points × rows × cols) so interp1 works on 1st dim

if abs(u) < 40

    A_lon = ...
        [-0.00894644618554263	0.0320555490226915	-1.19654303458228	-9.78886874671681;
0.0177938328871363	-2.75625714952099	41.9669994347238	0.0565348232672847;
0.00544480361520019	0.0390031290231026	-1.68547625422026	0;
0	0	0.999701937133157	0];
    B_lon = ...
        [-2.10906781602821	-8.34051477693776	-0.000966485101117076;
-228.851268194816	-60.5903363544424	-2.65783402805475;
-7.49489399091787	-17.9234263896394	-1.11495618916578;
0	0	0];

else

    u = abs(u);
    u = min(max(u, min(U)), max(U));

    A_lon =  squeeze( interp1(U, permute(A_lon_all,[3 1 2]), u, method, 'extrap') );
    B_lon =  squeeze( interp1(U, permute(B_lon_all,[3 1 2]), u, method, 'extrap') );

end

%% 3 Output
x_dot_lon = A_lon * x_lon + B_lon * u_lon;

end

== matlab function Longitudinal_U/Pitch-Attitude Hold/Controller variable ==
  data: Kp output; u input; Ki output
function [Kp, Ki] = Find_K2(u)
% Author:
%   Hanchen Li (hl3422@ic.ac.uk)
%
% Inputs:
%   u         - Forward velocity (m/s)
%
% Outputs:
%  Kp

U = [10.01; 20; 40; 60; 72.0222222];

if abs(u) <= 40

    Kp = -9.83;

    Ki = -0.010;

else
    
    u = abs(u);

    
    Kp_s = [-51.2 -43.4 -9.83 -5.57 -3.57];

    Ki_s = [-0.055 -0.043 -0.010 -0.020 -0.017];
    
    Kp =  interp1(U, Kp_s, u, 'pchip', 'extrap');
    
    Ki =  interp1(U, Ki_s, u, 'pchip', 'extrap');
    
end

end

== matlab function Longitudinal_U/Pitch Trim/Controller variable ==
  data: Kp output; u input; Ki output
function [Kp, Ki] = Find_K3(u)
% Author:
%   Hanchen Li (hl3422@ic.ac.uk)
%
% Inputs:
%   u         - Forward velocity (m/s)
%
% Outputs:
%  Kp

U = [10.01; 20; 40; 60; 72.0222222];

if abs(u) <= 10

    Kp = -0.033;

    Ki = -0.00020;

else

    u = abs(u);
    u = min(max(u, min(U)), max(U));
    
    Kp_s = [-0.057 -0.057 -0.033 -0.023 -0.023];

    Ki_s = [-0.0003 -0.00020 -0.00020 -0.000019 -0.000019];
    
    Kp =  interp1(U, Kp_s, u, 'pchip', 'extrap');
    
    Ki =  interp1(U, Ki_s, u, 'pchip', 'extrap');

end

end

== matlab function Longitudinal_U/Vertical Velocity Hold/Controller variable ==
  data: Kp output; u input; Ki output
function [Kp, Ki] = Find_K4(u)
% Author:
%   Hanchen Li (hl3422@ic.ac.uk)
%
% Inputs:
%   u         - Forward velocity (m/s)
%
% Outputs:
%  Kp

U = [10.01; 20; 40; 60; 72.0222222];

if abs(u) <= 40

    Kp = -0.0015;

    Ki = -0.0052;

else

    u = abs(u);
    u = min(max(u, min(U)), max(U));
    
    Kp_s = [-0.00045 -0.00045 -0.0015 -0.0015 -0.0015];

    Ki_s = [-0.0022 -0.0022 -0.0052 -0.0065 -0.0085];
    
    Kp =  interp1(U, Kp_s, u, 'pchip', 'extrap');
    
    Ki =  interp1(U, Ki_s, u, 'pchip', 'extrap');
    
end

end

== matlab function Longitudinal_U/Blend Factor ==
  data: blend output; u input
function blend = Blend_pitch(u)
% Author:
%   Hanchen Li (hl3422@ic.ac.uk)
%
% Inputs:
%   u         - Forward velocity (m/s)
%
% Outputs:
%   blend     - blend factor

%% 1 Decide blend factor

if abs(u) < 1e-4

    blend = 0;

elseif abs(u) < 90.3

    blend = u / (90.3 / 0.8);

else

    blend = 0.8;

end

end

== matlab function Longitudinal_U/Altitude Hold/Controller variable ==
  data: Kp output; u input; Ki output
function [Kp, Ki] = Find_K4(u)
% Author:
%   Hanchen Li (hl3422@ic.ac.uk)
%
% Inputs:
%   u         - Forward velocity (m/s)
%
% Outputs:
%  Kp

U = [10.01; 20; 40; 60; 72.0222222];

if abs(u) <= 40

    Kp = -0.13;

    Ki = -0.000017;

else

    u = abs(u);
    u = min(max(u, min(U)), max(U));
    
    Kp_s = [-0.13 -0.13 -0.15 -0.15 -0.15];

    Ki_s = [-0.000017 -0.000017 -0.000017 -0.000017 -0.000017];
    
    Kp =  interp1(U, Kp_s, u, 'pchip', 'extrap');
    
    Ki =  interp1(U, Ki_s, u, 'pchip', 'extrap');
    
end

end
